simulink model "lab_7_simulink"  (R2024b)
settings: Solver=ode45  StartTime=0.0  StopTime=15  MaxStep=1/32  RelTol=1e-3
settings Model: Creator=lw53894  LastModifiedBy=lw53894

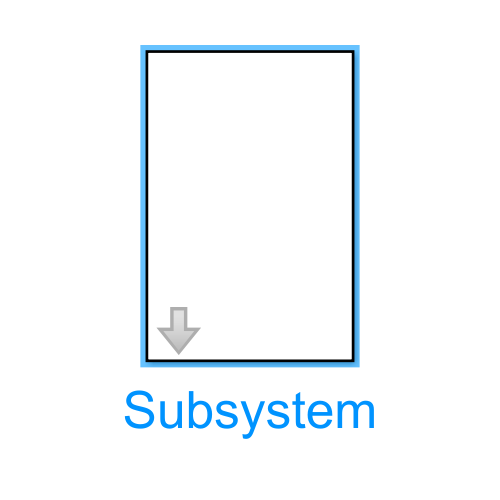
[thumbnail: Simulink's stored preview of the top-level diagram]
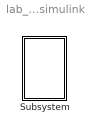
== system lab_7_simulink ==
  Subsystem : Subsystem  mask{g=9.81, k1=2, k2=1, m1=1, m2=2, l1=1, l2=2, fi1=80, fi2=150, fi_1_prim=0, fi_2_prim=0}

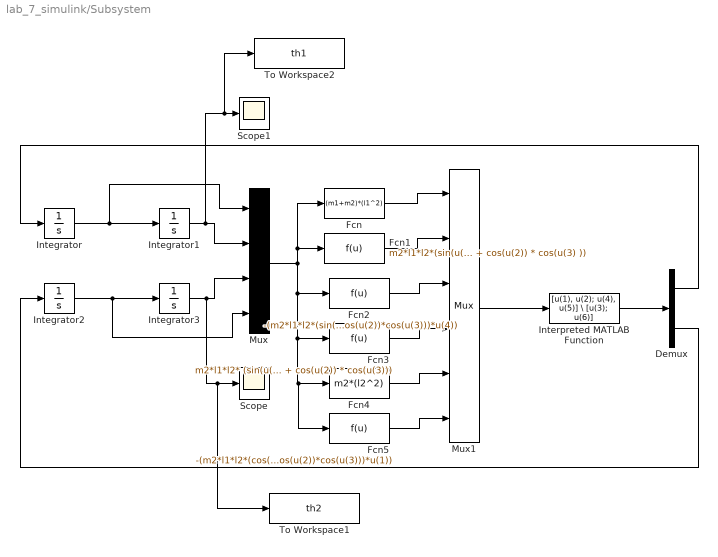
== system lab_7_simulink/Subsystem ==
  Demux : Demux  Outputs=2
  Fcn : Fcn  Expr=(m1+m2)*(l1^2)
  Fcn1 : Fcn  Expr=m2*l1*l2*(sin(u(2)) * sin(u(3)) + cos(u(2)) * cos(u(3) ))
  Fcn2 : Fcn  Expr=-(m2*l1*l2*(sin(u(2))*cos(u(3))-cos(u(2))*sin(u(3)))*u(4)^2+(m1+m2)*g*l1*sin(u(2))+k1*l1^2*u(1)+k2*l1*l2*(sin(u(2))*sin(u(3))+cos(u(2))*cos(u(3)))*u(4))
  Fcn3 : Fcn  Expr=m2*l1*l2* (sin(u(2)) * sin(u(3)) + cos(u(2)) * cos(u(3)))
  Fcn4 : Fcn  Expr=m2*(l2^2)
  Fcn5 : Fcn  Expr=-(m2*l1*l2*(cos(u(2))*sin(u(3))-sin(u(2))*cos(u(3)))*u(1)^2+m2*g*l2*sin(u(3))+k2*l2^2*u(4)+k2*l1*l2*(sin(u(2))*sin(u(3))+cos(u(2))*cos(u(3)))*u(1))
  Integrator : Integrator  InitialCondition=(fi_1_prim*pi)/180
  Integrator1 : Integrator  InitialCondition=(fi1*pi)/180
  Integrator2 : Integrator  InitialCondition=(fi_2_prim*pi)/180
  Integrator3 : Integrator  InitialCondition=(fi2*pi)/180
  Interpreted MATLAB Function : MATLABFcn  MATLABFcn=[u(1), u(2); u(4), u(5)] \ [u(3); u(6)]
  Mux : Mux
  Mux1 : Mux  Inputs=6
  Scope : Scope
  Scope1 : Scope
  To Workspace1 : ToWorkspace  VariableName=th2  SampleTime=-1
  To Workspace2 : ToWorkspace  VariableName=th1  SampleTime=-1
  wires:
  Interpreted MATLAB Function/1 -> Demux/1
  Mux/1 -> Fcn1/1, Fcn/1, Fcn5/1, Fcn4/1, Fcn3/1, Fcn2/1
  Integrator/1 -> Mux/1, Integrator1/1
  Integrator2/1 -> Mux/4, Integrator3/1
  Demux/2 -> Integrator2/1
  Fcn3/1 -> Mux1/4
  Fcn2/1 -> Mux1/3
  Integrator1/1 -> To Workspace2/1, Scope1/1, Mux/2
  Fcn5/1 -> Mux1/6
  Fcn4/1 -> Mux1/5
  Fcn/1 -> Mux1/1
  Integrator3/1 -> To Workspace1/1, Scope/1, Mux/3
  Fcn1/1 -> Mux1/2
  Mux1/1 -> Interpreted MATLAB Function/1
  Demux/1 -> Integrator/1
